simulink model "phase_shifter"  (R2015a)
settings: Solver=ode45  StartTime=0.0  StopTime=1e-8  FixedStep=200e-15  MaxStep=200e-15  MinStep=50e-15  RelTol=1e-3
libraries: SiPhotonics x2
settings Model: Creator=lins08  LastModifiedBy=lins08
settings SolverCC: InitialStep=50e-15

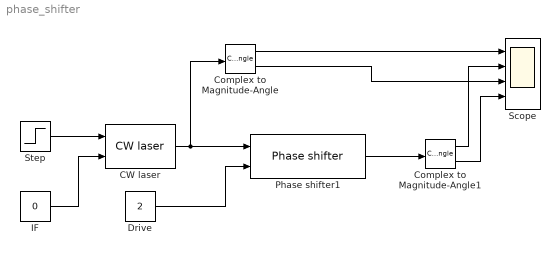
== system phase_shifter ==
  CW laser : SiPhotonics/CW laser
  Complex to Magnitude-Angle : ComplexToMagnitudeAngle
  Complex to Magnitude-Angle1 : ComplexToMagnitudeAngle
  Drive : Constant  Value=2
  IF : Constant  Value=0
  Phase shifter1 : SiPhotonics/Phase shifter  L=3e-3  fref=230e12  n0=2  ng=3  a0=300  c0=3e8  n1=8e-5  a1=-0.3  Ne=5e17  Nh=5e17  Vbi=0.7  Lj=0.5e-4  f0=230e12  opt=diode model
  Scope : Scope  NumInputPorts=4
      settings: YMin=-5~-5~-5~-5  YMax=5~5~5~5  MaxDataPoints=50000
  Step : Step  Time=1e-9  SampleTime=0
  wires:
  CW laser/1 -> Phase shifter1/1, Complex to Magnitude-Angle/1
  Drive/1 -> Phase shifter1/2
  Complex to Magnitude-Angle/1 -> Scope/1
  Complex to Magnitude-Angle1/2 -> Scope/4
  Phase shifter1/1 -> Complex to Magnitude-Angle1/1
  IF/1 -> CW laser/2
  Step/1 -> CW laser/1
  Complex to Magnitude-Angle1/1 -> Scope/2
  Complex to Magnitude-Angle/2 -> Scope/3
